simulink model "half_wave"  (R2024b)
settings: Solver=VariableStepAuto  StartTime=0.0  StopTime=10.0  RelTol=1e-3
values from neighbouring files (symbols this model uses):
  alpha_1_t = alpha_rad/(2*pi*f)    [simulink_params.m]
  f = double(f)    [ChargeFWR.m]    (also in full_wave_rectifier_CT.m = @(xx) arrayfun(@(xval) compute_power_loss(xval, alpha, beta,; simulink_params.m = 50)
  R = 20    [simulink_params.m]
  Vin_peak = sqrt(2)*Vin_rms    [simulink_params.m]
libraries: spsVoltageMeasurementLib x3, spsACVoltageSourceLib x1, spsCurrentMeasurementLib x1, spsMeanPhasorLib x1, spsSeriesRLCBranchLib x1, spsThyristorLib x1, sps_lib x1
settings Model: Creator=George  LastModifiedBy=George
settings DataIOCC: ExternalInput=[f, alpha_rad]

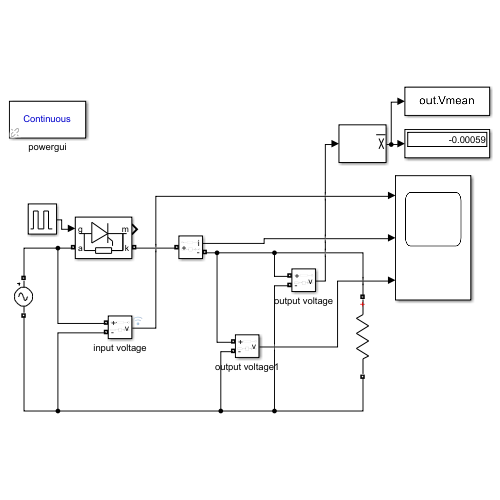
[thumbnail: Simulink's stored preview of the top-level diagram]
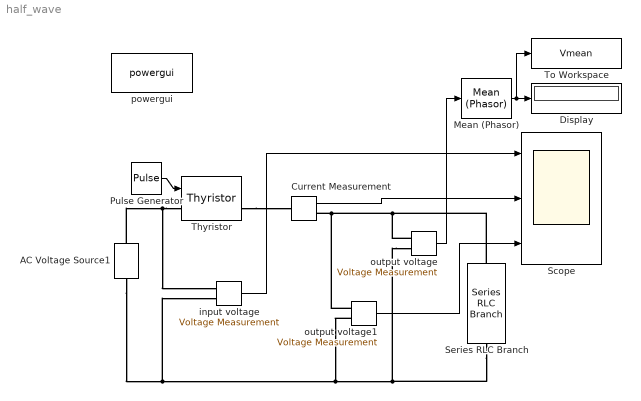
== system half_wave ==
  AC Voltage Source1 : spsACVoltageSourceLib/AC Voltage Source  Amplitude=Vin_peak  Phase=0  Frequency=f  SampleTime=0  Measurements=None  BusType=swing  Pref=10e3  Qref=0  Qmin=-inf  Qmax=+inf
  Current Measurement : spsCurrentMeasurementLib/Current Measurement  PhasorSimulation=off  OutputType=Complex  PSBequivalent=0
  Display : Display
  Mean (Phasor) : spsMeanPhasorLib/Mean (Phasor)  Freq=f  Vinit=0  Ts=0
      settings: LibrarySourceBlock=|
      | sps_lib/Sensors and Measurements/Mean
      | (Phasor)
  Pulse Generator : DiscretePulseGenerator  PulseType=Time based  Amplitude=2  Period=1/f  PulseWidth=5  PhaseDelay=alpha_1_t
  Scope : Scope  NumInputPorts=3
  Series RLC Branch : spsSeriesRLCBranchLib/Series RLC Branch  LConnTagsString=__new0  RConnTagsString=__new0  BranchType=R  Resistance=R  Inductance=0.1  SetiL0=off  InitialCurrent=0  Capacitance=0  Setx0=off  InitialVoltage=0  Measurements=None
  Thyristor : spsThyristorLib/Thyristor  Ron=0.001  Lon=0  Vf=0.75  IC=0  Rs=500  Cs=250e-6  Measurements=on
  To Workspace : ToWorkspace  VariableName=Vmean  SampleTime=-1
  input voltage : spsVoltageMeasurementLib/Voltage Measurement  PhasorSimulation=off  OutputType=Complex  PSBequivalent=0
  output voltage : spsVoltageMeasurementLib/Voltage Measurement  PhasorSimulation=off  OutputType=Complex  PSBequivalent=0
  output voltage1 : spsVoltageMeasurementLib/Voltage Measurement  PhasorSimulation=off  OutputType=Complex  PSBequivalent=0
  powergui : sps_lib/powergui  Priority=1  SimulationMode=Continuous  SampleTime=50e-6  frequency=50  Iterations=50  frequencyindice=50  Pbase=100e6  ErrMax=1e-4  UnitsV=kV  UnitsW=MW  buscounter=0  FunctionMessages=off  echomessages=off  EnableUseOfTLC=off  CurrentSourceSwitches=off  DisableSnubberDevices=off  DisableRonSwitches=off  DisableVfSwitches=off  DisplayEquations=off  AutomaticDiscreteSolvers=off  SolverType=Tustin/Backward Euler (TBE)  Interpol=off  ExternalGateDelay=off  methode=off  Ts=100  x0status=blocks  SPID=on  SwTol=0  HookPort=off  NonlinearTolerance=1e-4  nMaxIteration=100  ContinueOnMaxIteration=off  RestoreLinks=warning  ResistiveCurrentMeasurement=off  Frange=[0:2:500]  Ylog=off  Xlog=on  ShowGrid=off  save=off  variable=ZData  structure=0  ZoomFFT=off  StartTime=0.0  cycles=1  DisplayStyle=1  fundamental=60  FreqAxis=off  MaxFrequency=1000  frequencyindicesteady=1  RmsSteady=1  display=off
  wires:
  input voltage/1 -> Scope/1
  Pulse Generator/1 -> Thyristor/1
  Current Measurement/1 -> Scope/2
  output voltage/1 -> Mean (Phasor)/1
  output voltage1/1 -> Scope/3
  Mean (Phasor)/1 -> To Workspace/1, Display/1
  connections:
  output voltage/LConn1 -- Series RLC Branch/LConn1 -- output voltage1/LConn1 -- Current Measurement/RConn1
  Thyristor/LConn1 -- input voltage/LConn1 -- AC Voltage Source1/RConn1
  output voltage/LConn2 -- output voltage1/LConn2 -- AC Voltage Source1/LConn1 -- input voltage/LConn2 -- Series RLC Branch/RConn1
  Thyristor/RConn1 -- Current Measurement/LConn1
